simulink model "SMCLotkaVolterraModel"  (R2018b)
settings: Solver=VariableStepAuto  StartTime=0.0  StopTime=20  RelTol=1e-3
values from neighbouring files (symbols this model uses):
  a = 3    [SMC_LV.m]    (also in SlidingModeControl.m)
  alpha1 = 0.025    [SMC_LV.m]
  alpha2 = 0.025    [SMC_LV.m]
  alpha3 = 0.025    [SMC_LV.m]
  b = 3    [SMC_LV.m]    (also in SlidingModeControl.m)
  c = 2    [SMC_LV.m]    (also in SlidingModeControl.m)
  delta_1 = 0.1    [SMC_LV.m]
  delta_2 = 0.02    [SMC_LV.m]
  delta_3 = 0.2    [SMC_LV.m]
  gamma1 = 0.1    [SMC_LV.m]
  gamma2 = 0.05    [SMC_LV.m]
  gamma3 = 0.05    [SMC_LV.m]
  Ini = [1.2; 1.2; 1.2]    [SMC_LV.m]    (also in SlidingModeControl.m)
  k1 = 90    [SMC_LV.m]
  k2 = 150    [SMC_LV.m]
  k3 = 80    [SMC_LV.m]
  lamda1 = 0.5    [SMC_LV.m]
  lamda2 = 0.5    [SMC_LV.m]
  lamda3 = 0.5    [SMC_LV.m]
  p_1 = 0.1    [SMC_LV.m]
  p_2 = 0.2    [SMC_LV.m]
  p_3 = 0.3    [SMC_LV.m]
  pert_a = 0.05    [SMC_LV.m]
  pert_b = 0.1    [SMC_LV.m]
  pert_c = 0.1    [SMC_LV.m]
  theta_1 = 0.1    [SMC_LV.m]
  theta_2 = 0.2    [SMC_LV.m]
  theta_3 = 0.2    [SMC_LV.m]
settings Model: Creator=user  LastModifiedBy=user

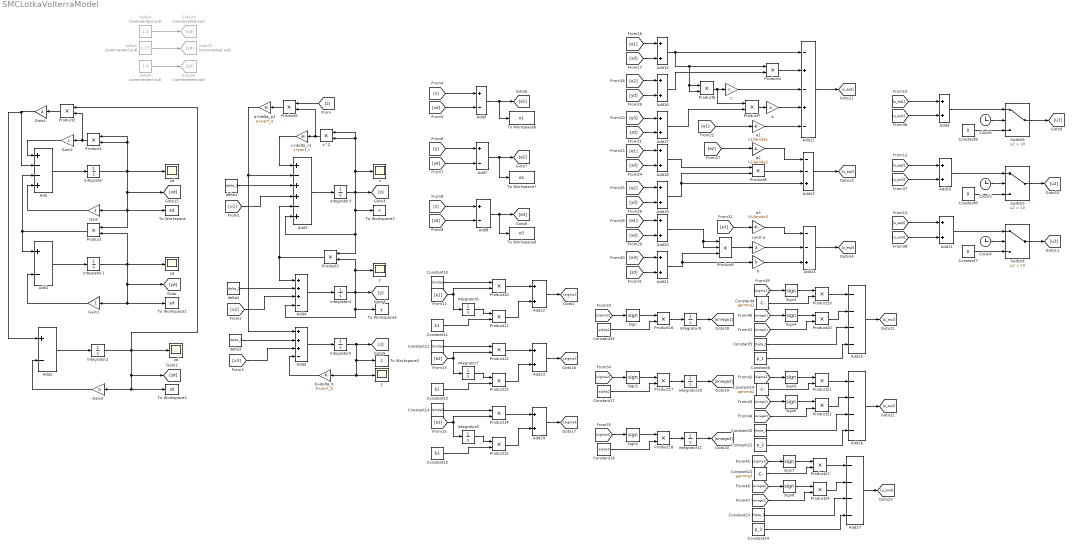
== system SMCLotkaVolterraModel ==
  Add : Sum  Inputs=+--+
  Add{1..2,6..8} (5 alike) : Sum  Inputs=+-
  Add{9..11,15..24} (13 alike) : Sum
  Add12 : Sum  Inputs=-+-+-
  Add13 : Sum  Inputs=--+
  Add14 : Sum  Inputs=--+
  Add25 : Sum  Inputs=----
  Add26 : Sum  Inputs=----
  Add27 : Sum  Inputs=----
  Add3 : Sum  Inputs=+-++-+
  Add4 : Sum  Inputs=+++-
  Add5 : Sum  Inputs=+++-
  Clock4 : Clock
  Clock5 : Clock
  Clock6 : Clock
  Constant10 : Constant  Value=lamda1
  Constant11 : Constant  Value=k1
  Constant12 : Constant  Value=lamda2
  Constant13 : Constant  Value=k2
  Constant14 : Constant  Value=lamda3
  Constant15 : Constant  Value=k3
  Constant16 : Constant  Value=alpha1
  Constant17 : Constant  Value=alpha2
  Constant18 : Constant  Value=alpha3
  Constant19 : Constant  Value=gamma2
  Constant20 : Constant  Value=theta_2
  Constant21 : Constant  Value=p_2
  Constant22 : Constant  Value=gamma3
  Constant23 : Constant  Value=theta_3
  Constant24 : Constant  Value=p_3
  Constant4 : Constant  Value=gamma1
  Constant5 : Constant  Value=theta_1
  Constant6 : Constant  Value=p_1
  Constant7 : Constant  Value=0
  Constant8 : Constant  Value=0
  Constant9 : Constant  Value=0
  Gain : Gain
  Gain1 : Gain
  Gain2 : Gain  Gain=c
  Gain3 : Gain  Gain=b
  Gain4 : Gain  Gain=a
  Goto24 : Goto  Commented=on  GotoTag=xd
  Goto25 : Goto  Commented=on  GotoTag=yd
  Goto26 : Goto  Commented=on  GotoTag=zd
  Integrator : Integrator  InitialCondition=Ini(1,1)
  Integrator1 : Integrator  InitialCondition=Ini(2,1)
  Integrator{6..11} (6 alike) : Integrator
  Integrator2 : Integrator  InitialCondition=Ini(3,1)
  Integrator3 : Integrator  InitialCondition=Ini(1,1)
  Integrator4 : Integrator  InitialCondition=Ini(2,1)
  Integrator5 : Integrator  InitialCondition=Ini(3,1)
  Product{,1..8,10..24} (24 alike) : Product
  Product9 : Product  Inputs=3
  Sign{,1..8} (9 alike) : Signum
  Switch4 : Switch  Criteria=u2 > Threshold  Threshold=10
  Switch5 : Switch  Criteria=u2 > Threshold  Threshold=10
  Switch6 : Switch  Criteria=u2 > Threshold  Threshold=10
  To Workspace : ToWorkspace  VariableName=xd  SampleTime=0.01
  To Workspace1 : ToWorkspace  VariableName=yd  SampleTime=0.01
  To Workspace2 : ToWorkspace  VariableName=zd  SampleTime=0.01
  To Workspace3 : ToWorkspace  VariableName=x  SampleTime=0.01
  To Workspace4 : ToWorkspace  VariableName=y  SampleTime=0.01
  To Workspace5 : ToWorkspace  VariableName=z  SampleTime=0.01
  To Workspace6 : ToWorkspace  VariableName=e1  SampleTime=-1
  To Workspace7 : ToWorkspace  VariableName=e2  SampleTime=-1
  To Workspace8 : ToWorkspace  VariableName=e3  SampleTime=-1
  a : Gain  Gain=a
  a+delta_a1 : Gain  Gain=a+pert_a
  a1 : Gain  Gain=k1/lamda1
  a2 : Gain  Gain=k2/lamda2
  a3 : Gain  Gain=k3/lamda3
  b : Gain  Gain=b
  b+delta_b : Gain  Gain=b+pert_b
  c : Gain  Gain=c
  c+delta_c1 : Gain  Gain=c+pert_c
  const a : Gain  Gain=a
  delta1 : Constant  Value=delta_1
  delta2 : Constant  Value=delta_2
  delta3 : Constant  Value=delta_3
  delta4 : Constant  Commented=on  Value=1.2
  delta5 : Constant  Commented=on  Value=1.15
  delta6 : Constant  Commented=on  Value=1.4
  x : Scope
  x^2 : Product
  xd : Scope
  y : Scope
  yd : Scope
  z : Scope
  zd : Scope
  wires:
  Product1/1 -> Product2/2, Gain2/1
  Gain3/1 -> Add2/2
  Add1/1 -> Integrator1/1
  Add2/1 -> Integrator2/1
  Gain1/1 -> Add1/2
  Product/1 -> Add1/1, Add/3
  Gain2/1 -> Add/1
  Gain4/1 -> Add2/1, Add/2
  Gain/1 -> Add/4
  Integrator/1 -> Product1/1, Product1/2, [xd], To Workspace/1, Product/1, Gain/1, xd/1
  Product2/1 -> Gain4/1
  Add/1 -> Integrator/1
  Add3/1 -> Integrator3/1
  Integrator3/1 -> x/1, x^2/1, x^2/2, To Workspace3/1, Add3/6, Product3/1, [x]
  Add4/1 -> Integrator4/1
  Add5/1 -> Integrator5/1
  Integrator5/1 -> z/1, b+delta_b/1, To Workspace5/1, [z]
  Integrator4/1 -> [y], To Workspace4/1, Add4/4, y/1, Product3/2
  x^2/1 -> c+delta_c1/1, Product5/2
  c+delta_c1/1 -> Add3/1
  Product5/1 -> a+delta_a1/1
  [z] -> Product5/1
  a+delta_a1/1 -> Add5/1, Add3/2
  Product3/1 -> Add4/1, Add3/5
  delta1/1 -> Add3/3
  [u1] -> Add3/4
  delta2/1 -> Add4/2
  [u2] -> Add4/3
  b+delta_b/1 -> Add5/4
  delta3/1 -> Add5/2
  [u3] -> Add5/3
  [x] -> Add6/1
  [y] -> Add7/1
  [z] -> Add8/1
  [u_eq3] -> Add11/1
  [u_eq2] -> Add10/1
  [u_eq1] -> Add9/1
  Add12/1 -> [u_eq1]
  Add13/1 -> [u_eq2]
  Add14/1 -> [u_eq3]
  [e1] -> Add15/1
  Add15/1 -> Product4/1, Product6/1, Product6/2, Add12/1
  [e2] -> Add16/1
  [e3] -> Add17/1
  Add16/1 -> Product4/2
  Product4/1 -> Add12/2
  c/1 -> Add12/3
  Product6/1 -> Product7/1, c/1
  a/1 -> Add12/4
  Product7/1 -> a/1
  Add17/1 -> Product7/2
  [e2] -> Add19/1
  [e1] -> Add18/1
  Add19/1 -> Product8/2, Add13/3
  Product8/1 -> Add13/2
  Add18/1 -> Product8/1
  [e1] -> Add20/1
  [e3] -> Add21/1
  b/1 -> Add14/3
  Add21/1 -> Product9/3, b/1
  Add20/1 -> Product9/2, Product9/1
  Product9/1 -> const a/1
  const a/1 -> Add14/2
  [e1] -> a1/1
  a1/1 -> Add12/5
  [e2] -> a2/1
  a2/1 -> Add13/1
  [e3] -> a3/1
  a3/1 -> Add14/1
  [xd] -> Add15/2
  [yd] -> Add16/2
  [zd] -> Add17/2
  [xd] -> Add18/2
  [yd] -> Add19/2
  [xd] -> Add20/2
  [zd] -> Add21/2
  [zd] -> Add8/2
  [yd] -> Add7/2
  Integrator1/1 -> [yd], To Workspace1/1, Gain1/1, Product/2, yd/1
  Integrator2/1 -> zd/1, Product2/1, [zd], To Workspace2/1, Gain3/1
  [xd] -> Add6/2
  Add6/1 -> To Workspace6/1, [e1]
  Add7/1 -> To Workspace7/1, [e2]
  Add8/1 -> To Workspace8/1, [e3]
  Constant7/1 -> Switch4/3
  Clock4/1 -> Switch4/2
  Add11/1 -> Switch4/1
  Switch4/1 -> [u3]
  Constant8/1 -> Switch5/3
  Switch5/1 -> [u2]
  Add10/1 -> Switch5/1
  Clock5/1 -> Switch5/2
  Clock6/1 -> Switch6/2
  Constant9/1 -> Switch6/3
  Switch6/1 -> [u1]
  Add9/1 -> Switch6/1
  Add22/1 -> [sigma1]
  Product10/1 -> Add22/1
  Constant10/1 -> Product10/1
  [e1] -> Product10/2, Integrator6/1
  Integrator6/1 -> Product11/1
  Constant11/1 -> Product11/2
  Product11/1 -> Add22/2
  Product13/1 -> Add23/2
  Constant13/1 -> Product13/2
  Integrator7/1 -> Product13/1
  [e2] -> Integrator7/1, Product12/2
  Constant12/1 -> Product12/1
  Product12/1 -> Add23/1
  Add23/1 -> [sigma2]
  Add24/1 -> [sigma3]
  Product14/1 -> Add24/1
  Constant14/1 -> Product14/1
  [e3] -> Product14/2, Integrator8/1
  Integrator8/1 -> Product15/1
  Constant15/1 -> Product15/2
  Product15/1 -> Add24/2
  [sigma1] -> Sign/1
  Sign/1 -> Product16/1
  Constant16/1 -> Product16/2
  Product16/1 -> Integrator9/1
  Integrator9/1 -> [omega1]
  Integrator10/1 -> [omega2]
  Product17/1 -> Integrator10/1
  Constant17/1 -> Product17/2
  Sign1/1 -> Product17/1
  [sigma2] -> Sign1/1
  [sigma3] -> Sign2/1
  Sign2/1 -> Product18/1
  Constant18/1 -> Product18/2
  Product18/1 -> Integrator11/1
  Integrator11/1 -> [omega3]
  [u_sw1] -> Add9/2
  [u_sw2] -> Add10/2
  [u_sw3] -> Add11/2
  Add25/1 -> [u_sw1]
  Constant4/1 -> Product19/2
  Sign3/1 -> Product19/1
  [sigma1] -> Sign3/1
  Product19/1 -> Add25/1
  [omega1] -> Sign4/1
  Sign4/1 -> Product20/1
  [omega1] -> Product20/2
  Product20/1 -> Add25/2
  Constant5/1 -> Add25/3
  Constant6/1 -> Add25/4
  Constant21/1 -> Add26/4
  Constant20/1 -> Add26/3
  Product22/1 -> Add26/2
  [omega2] -> Product22/2
  Sign6/1 -> Product22/1
  [omega2] -> Sign6/1
  Product21/1 -> Add26/1
  [sigma2] -> Sign5/1
  Sign5/1 -> Product21/1
  Constant19/1 -> Product21/2
  Add26/1 -> [u_sw2]
  Add27/1 -> [u_sw3]
  Constant22/1 -> Product23/2
  Sign7/1 -> Product23/1
  [sigma3] -> Sign7/1
  Product23/1 -> Add27/1
  [omega3] -> Sign8/1
  Sign8/1 -> Product24/1
  [omega3] -> Product24/2
  Product24/1 -> Add27/2
  Constant23/1 -> Add27/3
  Constant24/1 -> Add27/4
  delta4/1 -> Goto24/1
  delta5/1 -> Goto25/1
  delta6/1 -> Goto26/1
